simulink model "TVCVehicleModelAndSimulation_SubsystemVersion"  (R2024a)
settings: Solver=VariableStepAuto  StartTime=0.0  StopTime=10.0  RelTol=1e-3
values from neighbouring files (symbols this model uses):
  Thrust_Moment_Arm = 0.1    [ModelVariables.m]
libraries: simulink_extras x2, shared6dof x1
settings Model: Creator=Joshua Caratao  LastModifiedBy=Joshua Caratao

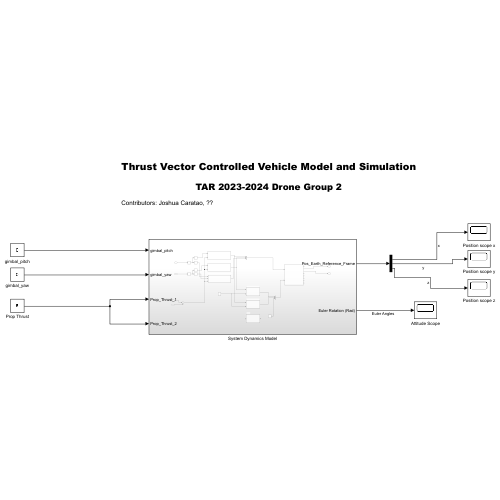
[thumbnail: Simulink's stored preview of the top-level diagram]
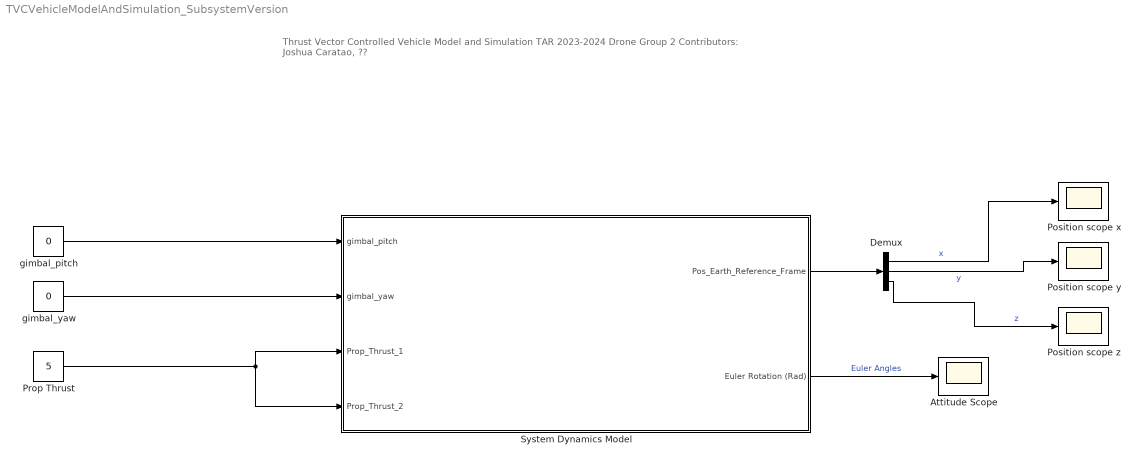
== system TVCVehicleModelAndSimulation_SubsystemVersion ==
  note: Thrust Vector Controlled Vehicle Model and Simulation
      |
      | TAR 2023-2024 Drone Group 2
      |
      | Contributors: Joshua Caratao, ??
  Attitude Scope : Scope
  Demux : Demux  Outputs=3
  Position scope x : Scope
  Position scope y : Scope
  Position scope z : Scope
  Prop Thrust : Constant  Value=5
  System Dynamics Model : Subsystem
  gimbal_pitch : Constant  Value=0
  gimbal_yaw : Constant  Value=0
  wires:
  Prop Thrust/1 -> System Dynamics Model/4(Prop_Thrust_2), System Dynamics Model/3(Prop_Thrust_1)
  gimbal_yaw/1 -> System Dynamics Model/2(gimbal_yaw)
  gimbal_pitch/1 -> System Dynamics Model/1(gimbal_pitch)
  System Dynamics Model/2(Euler Rotation (Rad)) -> Attitude Scope/1  "Euler Angles"
  System Dynamics Model/1(Pos_Earth_Reference_Frame) -> Demux/1
  Demux/1 -> Position scope x/1  "x"
  Demux/2 -> Position scope y/1  "y"
  Demux/3 -> Position scope z/1  "z"

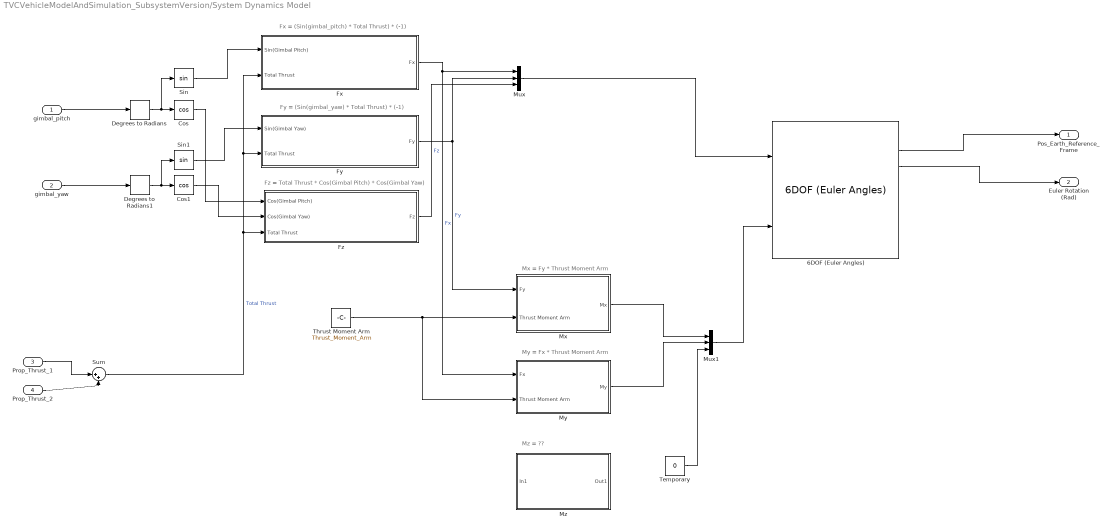
== system TVCVehicleModelAndSimulation_SubsystemVersion/System Dynamics Model ==
  note: Fx = (Sin(gimbal_pitch) * Total Thrust) * (-1)
  note: Fy = (Sin(gimbal_yaw) * Total Thrust) * (-1)
  note: Fz = Total Thrust * Cos(Gimbal Pitch) * Cos(Gimbal Yaw)
  note: My = Fx * Thrust Moment Arm
  note: Mx = Fy * Thrust Moment Arm
  note: Mz = ??
  gimbal_pitch : Inport
  gimbal_yaw : Inport  Port=2
  Prop_Thrust_1 : Inport  Port=3
  Prop_Thrust_2 : Inport  Port=4
  6DOF (Euler Angles) : shared6dof/6DOF (Euler Angles)  units=Metric (MKS)  mtype=Fixed  rep=Euler Angles  xme_0=Initial_Pos_Inertial_Axes  Vm_0=Initial_Vel_Body_Axes  eul_0=Initial_Euler_Orientation  pm_0=Initial_Body_Rotation_Rates  mass_0=Mass  mass_e=0.5  mass_f=2.0  inertia=Inertia_Tensor  inertia_e=eye(3)  inertia_f=2*eye(3)  k_quat=1.0  vre_flag=on  abi_flag=off  aMode=0  xme_statename=''  Vm_statename=''  eul_statename=''  quat_statename=''  pm_statename=''  mass_statename=''
  Cos : Trigonometry  Operator=cos
  Cos1 : Trigonometry  Operator=cos
  Degrees to Radians : simulink_extras/Transformations/Degrees to Radians
  Degrees to Radians1 : simulink_extras/Transformations/Degrees to Radians
  Fx : Subsystem
  Fy : Subsystem
  Fz : Subsystem
  Mux : Mux  Inputs=3
  Mux1 : Mux  Inputs=3
  Mx : Subsystem
  My : Subsystem
  Mz : Subsystem
  Sin : Trigonometry
  Sin1 : Trigonometry
  Sum : Sum  Inputs=|++
  Temporary : Constant  Value=0
  "Thrust Moment Arm " : Constant  Value=Thrust_Moment_Arm
  Pos_Earth_Reference_Frame : Outport
  Euler Rotation (Rad) : Outport  Port=2
  wires:
  Mux1/1 -> 6DOF (Euler Angles)/2
  Mux/1 -> 6DOF (Euler Angles)/1
  gimbal_pitch/1 -> Degrees to Radians/1
  gimbal_yaw/1 -> Degrees to Radians1/1
  Degrees to Radians/1 -> Sin/1, Cos/1
  Degrees to Radians1/1 -> Sin1/1, Cos1/1
  Prop_Thrust_1/1 -> Sum/1
  Prop_Thrust_2/1 -> Sum/2
  Sin/1 -> Fx/1(Sin(Gimbal Pitch))
  Sum/1 -> Fz/3(Total Thrust), Fx/2(Total Thrust), Fy/2(Total Thrust)  "Total Thrust"
  Fx/1(Fx) -> Mux/1, My/1(Fx)  "Fx"
  Sin1/1 -> Fy/1(Sin(Gimbal Yaw))
  Fy/1(Fy) -> Mux/2, Mx/1(Fy)  "Fy"
  Cos1/1 -> Fz/2(Cos(Gimbal Yaw))
  Cos/1 -> Fz/1(Cos(Gimbal Pitch))
  Fz/1(Fz) -> Mux/3  "Fz"
  "Thrust Moment Arm "/1 -> Mx/2(Thrust Moment Arm), My/2(Thrust Moment Arm)
  My/1(My) -> Mux1/2
  Mx/1(Mx) -> Mux1/1
  Temporary/1 -> Mux1/3
  6DOF (Euler Angles)/2 -> Pos_Earth_Reference_Frame/1
  6DOF (Euler Angles)/3 -> Euler Rotation (Rad)/1

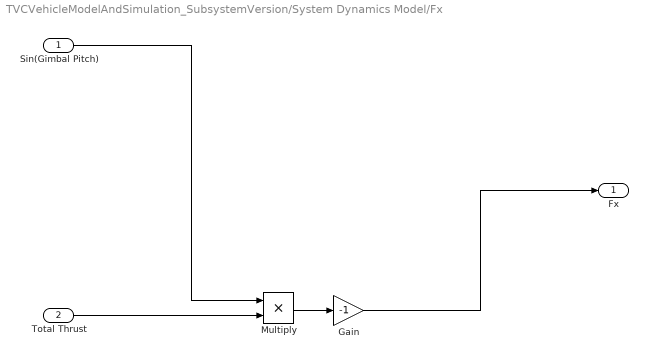
== system TVCVehicleModelAndSimulation_SubsystemVersion/System Dynamics Model/Fx ==
  Sin(Gimbal Pitch) : Inport
  Total Thrust : Inport  Port=2
  Gain : Gain  Gain=-1
  Multiply : Product
  Fx : Outport
  wires:
  Multiply/1 -> Gain/1
  Sin(Gimbal Pitch)/1 -> Multiply/1
  Total Thrust/1 -> Multiply/2
  Gain/1 -> Fx/1

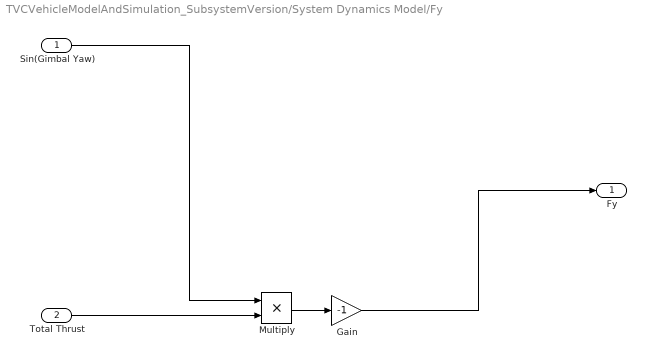
== system TVCVehicleModelAndSimulation_SubsystemVersion/System Dynamics Model/Fy ==
  Sin(Gimbal Yaw) : Inport
  Total Thrust : Inport  Port=2
  Gain : Gain  Gain=-1
  Multiply : Product
  Fy : Outport
  wires:
  Multiply/1 -> Gain/1
  Sin(Gimbal Yaw)/1 -> Multiply/1
  Total Thrust/1 -> Multiply/2
  Gain/1 -> Fy/1

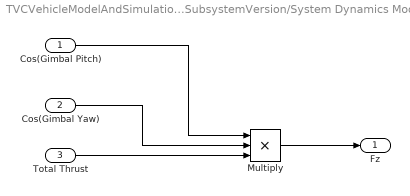
== system TVCVehicleModelAndSimulation_SubsystemVersion/System Dynamics Model/Fz ==
  Cos(Gimbal Pitch) : Inport
  Cos(Gimbal Yaw) : Inport  Port=2
  Total Thrust : Inport  Port=3
  Multiply : Product  Inputs=3
  Fz : Outport
  wires:
  Cos(Gimbal Pitch)/1 -> Multiply/1
  Cos(Gimbal Yaw)/1 -> Multiply/2
  Multiply/1 -> Fz/1
  Total Thrust/1 -> Multiply/3

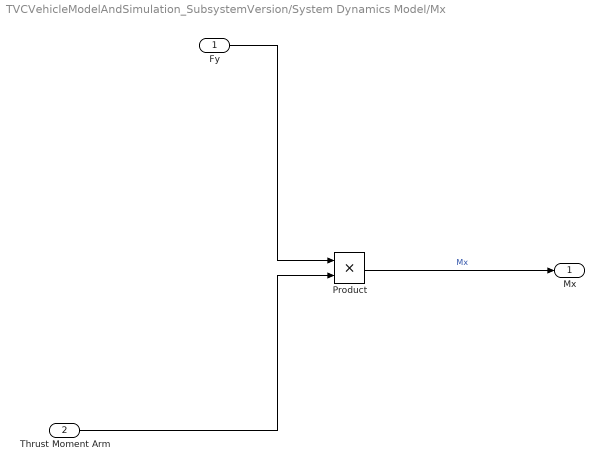
== system TVCVehicleModelAndSimulation_SubsystemVersion/System Dynamics Model/Mx ==
  Fy : Inport
  Thrust Moment Arm : Inport  Port=2
  Product : Product
  Mx : Outport
  wires:
  Thrust Moment Arm/1 -> Product/2
  Fy/1 -> Product/1
  Product/1 -> Mx/1  "Mx"

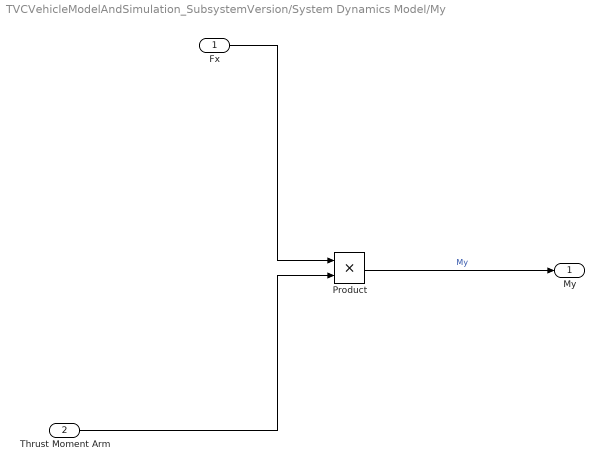
== system TVCVehicleModelAndSimulation_SubsystemVersion/System Dynamics Model/My ==
  Fx : Inport
  Thrust Moment Arm : Inport  Port=2
  Product : Product
  My : Outport
  wires:
  Thrust Moment Arm/1 -> Product/2
  Fx/1 -> Product/1
  Product/1 -> My/1  "My"

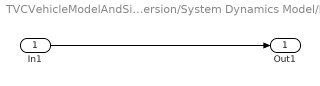
== system TVCVehicleModelAndSimulation_SubsystemVersion/System Dynamics Model/Mz ==
  In1 : Inport
  Out1 : Outport
  wires:
  In1/1 -> Out1/1
